simulink model "ALU_04_SS"  (R2022a)
settings: Solver=VariableStepAuto  StartTime=0.0  StopTime=10.0  RelTol=1e-3
undefined symbols (not defined in the file or in its folder): xc7z010iclg225
libraries: hdlBasic x1537, vmcUtilities x1
(part 3 of 8)

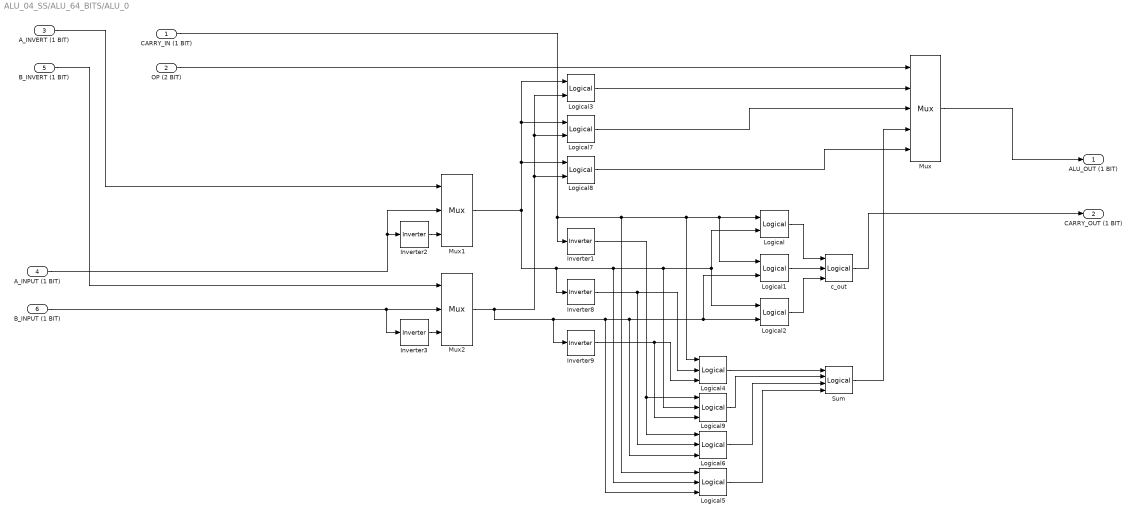
== system ALU_04_SS/ALU_64_BITS/ALU_0 ==
  CARRY_IN (1 BIT) : Inport
  OP (2 BIT) : Inport  Port=2
  A_INVERT (1 BIT) : Inport  Port=3
  A_INPUT (1 BIT) : Inport  Port=4
  B_INVERT (1 BIT) : Inport  Port=5
  B_INPUT (1 BIT) : Inport  Port=6
  Inverter{1..3,8..9} (5 alike) : hdlBasic/Inverter  en=off  latency=0  XmcBlockStatus=1  maskContainerNames=group2  block_type=inv  block_config=sysgen:Inverter_config
  Logical{,1..3} (4 alike) : hdlBasic/Logical  logical_function=AND  inputs=2  en=off  latency=0  precision=Full  arith_type=Unsigned  n_bits=16  bin_pt=0  align_bp=on  overflow=[]  quantization=[]  XmcBlockStatus=1  maskContainerNames=tabcontainer1  block_type=logical  block_config=sysgen:Logical_config
  Logical{4..6,9} (4 alike) : hdlBasic/Logical  logical_function=AND  inputs=3  en=off  latency=0  precision=Full  arith_type=Unsigned  n_bits=16  bin_pt=0  align_bp=on  overflow=[]  quantization=[]  XmcBlockStatus=1  maskContainerNames=tabcontainer1  block_type=logical  block_config=sysgen:Logical_config
  Logical7 : hdlBasic/Logical  logical_function=OR  inputs=2  en=off  latency=0  precision=Full  arith_type=Unsigned  n_bits=16  bin_pt=0  align_bp=on  overflow=[]  quantization=[]  XmcBlockStatus=1  maskContainerNames=tabcontainer1  block_type=logical  block_config=sysgen:Logical_config
  Logical8 : hdlBasic/Logical  logical_function=XOR  inputs=2  en=off  latency=0  precision=Full  arith_type=Unsigned  n_bits=16  bin_pt=0  align_bp=on  overflow=[]  quantization=[]  XmcBlockStatus=1  maskContainerNames=tabcontainer1  block_type=logical  block_config=sysgen:Logical_config
  Mux : hdlBasic/Mux  inputs=4  en=off  latency=0  precision=Full  arith_type=Unsigned  n_bits=16  bin_pt=14  quantization=Truncate  overflow=Wrap  XmcBlockStatus=1  maskContainerNames=tabcontainer1  block_type=mux  block_config=sysgen:Mux_config
  Mux1 : hdlBasic/Mux  inputs=2  en=off  latency=0  precision=Full  arith_type=Unsigned  n_bits=16  bin_pt=14  quantization=Truncate  overflow=Wrap  XmcBlockStatus=1  maskContainerNames=tabcontainer1  block_type=mux  block_config=sysgen:Mux_config
  Mux2 : hdlBasic/Mux  inputs=2  en=off  latency=0  precision=Full  arith_type=Unsigned  n_bits=16  bin_pt=14  quantization=Truncate  overflow=Wrap  XmcBlockStatus=1  maskContainerNames=tabcontainer1  block_type=mux  block_config=sysgen:Mux_config
  Sum : hdlBasic/Logical  logical_function=OR  inputs=4  en=off  latency=0  precision=Full  arith_type=Unsigned  n_bits=16  bin_pt=0  align_bp=on  overflow=[]  quantization=[]  XmcBlockStatus=1  maskContainerNames=tabcontainer1  block_type=logical  block_config=sysgen:Logical_config
  c_out : hdlBasic/Logical  logical_function=OR  inputs=3  en=off  latency=0  precision=Full  arith_type=Unsigned  n_bits=16  bin_pt=0  align_bp=on  overflow=[]  quantization=[]  XmcBlockStatus=1  maskContainerNames=tabcontainer1  block_type=logical  block_config=sysgen:Logical_config
  ALU_OUT (1 BIT) : Outport
  CARRY_OUT (1 BIT) : Outport  Port=2
  wires:
  Logical2/1 -> c_out/3
  A_INVERT (1 BIT)/1 -> Mux1/1
  c_out/1 -> CARRY_OUT (1 BIT)/1
  Sum/1 -> Mux/4
  CARRY_IN (1 BIT)/1 -> Inverter1/1, Logical5/1, Logical4/1, Logical1/1, Logical/1
  Mux2/1 -> Logical5/3, Logical6/3, Logical1/2, Logical2/2, Inverter9/1, Logical8/2, Logical3/2, Logical7/2
  B_INPUT (1 BIT)/1 -> Inverter3/1, Mux2/2
  Mux/1 -> ALU_OUT (1 BIT)/1
  Logical/1 -> c_out/1
  B_INVERT (1 BIT)/1 -> Mux2/1
  Logical6/1 -> Sum/3
  Mux1/1 -> Logical8/1, Logical7/1, Logical3/1, Inverter8/1, Logical5/2, Logical/2, Logical2/1, Logical9/2
  Logical5/1 -> Sum/4
  OP (2 BIT)/1 -> Mux/1
  Logical9/1 -> Sum/2
  Inverter1/1 -> Logical6/1, Logical9/1
  Inverter3/1 -> Mux2/3
  Inverter9/1 -> Logical9/3, Logical4/3
  A_INPUT (1 BIT)/1 -> Mux1/2, Inverter2/1
  Inverter2/1 -> Mux1/3
  Logical4/1 -> Sum/1
  Inverter8/1 -> Logical6/2, Logical4/2
  Logical3/1 -> Mux/2
  Logical7/1 -> Mux/3
  Logical1/1 -> c_out/2
  Logical8/1 -> Mux/5

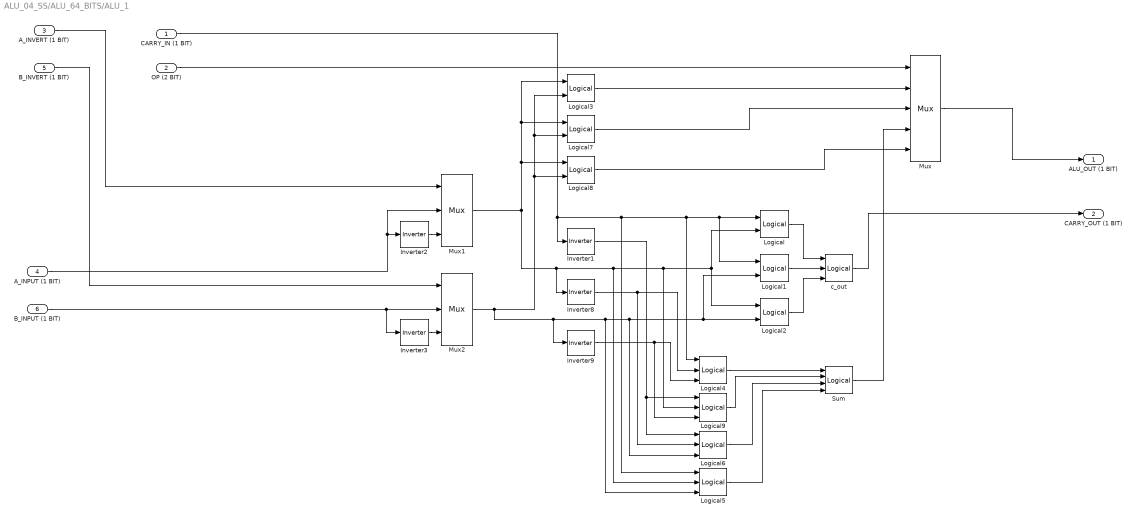
== system ALU_04_SS/ALU_64_BITS/ALU_1 ==
  CARRY_IN (1 BIT) : Inport
  OP (2 BIT) : Inport  Port=2
  A_INVERT (1 BIT) : Inport  Port=3
  A_INPUT (1 BIT) : Inport  Port=4
  B_INVERT (1 BIT) : Inport  Port=5
  B_INPUT (1 BIT) : Inport  Port=6
  Inverter{1..3,8..9} (5 alike) : hdlBasic/Inverter  en=off  latency=0  XmcBlockStatus=1  maskContainerNames=group2  block_type=inv  block_config=sysgen:Inverter_config
  Logical{,1..3} (4 alike) : hdlBasic/Logical  logical_function=AND  inputs=2  en=off  latency=0  precision=Full  arith_type=Unsigned  n_bits=16  bin_pt=0  align_bp=on  overflow=[]  quantization=[]  XmcBlockStatus=1  maskContainerNames=tabcontainer1  block_type=logical  block_config=sysgen:Logical_config
  Logical{4..6,9} (4 alike) : hdlBasic/Logical  logical_function=AND  inputs=3  en=off  latency=0  precision=Full  arith_type=Unsigned  n_bits=16  bin_pt=0  align_bp=on  overflow=[]  quantization=[]  XmcBlockStatus=1  maskContainerNames=tabcontainer1  block_type=logical  block_config=sysgen:Logical_config
  Logical7 : hdlBasic/Logical  logical_function=OR  inputs=2  en=off  latency=0  precision=Full  arith_type=Unsigned  n_bits=16  bin_pt=0  align_bp=on  overflow=[]  quantization=[]  XmcBlockStatus=1  maskContainerNames=tabcontainer1  block_type=logical  block_config=sysgen:Logical_config
  Logical8 : hdlBasic/Logical  logical_function=XOR  inputs=2  en=off  latency=0  precision=Full  arith_type=Unsigned  n_bits=16  bin_pt=0  align_bp=on  overflow=[]  quantization=[]  XmcBlockStatus=1  maskContainerNames=tabcontainer1  block_type=logical  block_config=sysgen:Logical_config
  Mux : hdlBasic/Mux  inputs=4  en=off  latency=0  precision=Full  arith_type=Unsigned  n_bits=16  bin_pt=14  quantization=Truncate  overflow=Wrap  XmcBlockStatus=1  maskContainerNames=tabcontainer1  block_type=mux  block_config=sysgen:Mux_config
  Mux1 : hdlBasic/Mux  inputs=2  en=off  latency=0  precision=Full  arith_type=Unsigned  n_bits=16  bin_pt=14  quantization=Truncate  overflow=Wrap  XmcBlockStatus=1  maskContainerNames=tabcontainer1  block_type=mux  block_config=sysgen:Mux_config
  Mux2 : hdlBasic/Mux  inputs=2  en=off  latency=0  precision=Full  arith_type=Unsigned  n_bits=16  bin_pt=14  quantization=Truncate  overflow=Wrap  XmcBlockStatus=1  maskContainerNames=tabcontainer1  block_type=mux  block_config=sysgen:Mux_config
  Sum : hdlBasic/Logical  logical_function=OR  inputs=4  en=off  latency=0  precision=Full  arith_type=Unsigned  n_bits=16  bin_pt=0  align_bp=on  overflow=[]  quantization=[]  XmcBlockStatus=1  maskContainerNames=tabcontainer1  block_type=logical  block_config=sysgen:Logical_config
  c_out : hdlBasic/Logical  logical_function=OR  inputs=3  en=off  latency=0  precision=Full  arith_type=Unsigned  n_bits=16  bin_pt=0  align_bp=on  overflow=[]  quantization=[]  XmcBlockStatus=1  maskContainerNames=tabcontainer1  block_type=logical  block_config=sysgen:Logical_config
  ALU_OUT (1 BIT) : Outport
  CARRY_OUT (1 BIT) : Outport  Port=2
  wires:
  Logical2/1 -> c_out/3
  A_INVERT (1 BIT)/1 -> Mux1/1
  c_out/1 -> CARRY_OUT (1 BIT)/1
  Sum/1 -> Mux/4
  CARRY_IN (1 BIT)/1 -> Inverter1/1, Logical5/1, Logical4/1, Logical1/1, Logical/1
  Mux2/1 -> Logical5/3, Logical6/3, Logical1/2, Logical2/2, Inverter9/1, Logical8/2, Logical3/2, Logical7/2
  B_INPUT (1 BIT)/1 -> Inverter3/1, Mux2/2
  Mux/1 -> ALU_OUT (1 BIT)/1
  Logical/1 -> c_out/1
  B_INVERT (1 BIT)/1 -> Mux2/1
  Logical6/1 -> Sum/3
  Mux1/1 -> Logical8/1, Logical7/1, Logical3/1, Inverter8/1, Logical5/2, Logical/2, Logical2/1, Logical9/2
  Logical5/1 -> Sum/4
  OP (2 BIT)/1 -> Mux/1
  Logical9/1 -> Sum/2
  Inverter1/1 -> Logical6/1, Logical9/1
  Inverter3/1 -> Mux2/3
  Inverter9/1 -> Logical9/3, Logical4/3
  A_INPUT (1 BIT)/1 -> Mux1/2, Inverter2/1
  Inverter2/1 -> Mux1/3
  Logical4/1 -> Sum/1
  Inverter8/1 -> Logical6/2, Logical4/2
  Logical3/1 -> Mux/2
  Logical7/1 -> Mux/3
  Logical1/1 -> c_out/2
  Logical8/1 -> Mux/5

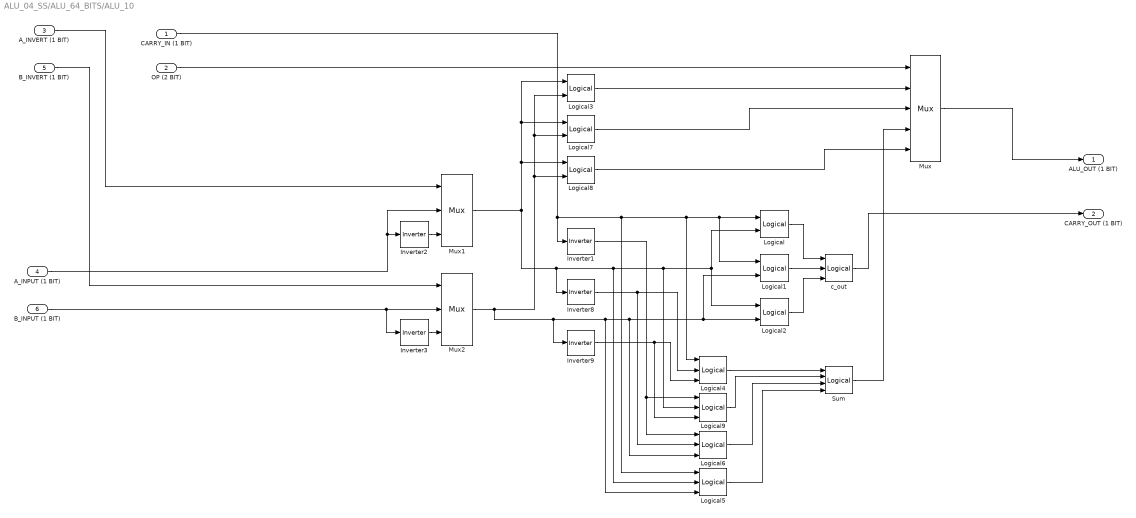
== system ALU_04_SS/ALU_64_BITS/ALU_10 ==
  CARRY_IN (1 BIT) : Inport
  OP (2 BIT) : Inport  Port=2
  A_INVERT (1 BIT) : Inport  Port=3
  A_INPUT (1 BIT) : Inport  Port=4
  B_INVERT (1 BIT) : Inport  Port=5
  B_INPUT (1 BIT) : Inport  Port=6
  Inverter{1..3,8..9} (5 alike) : hdlBasic/Inverter  en=off  latency=0  XmcBlockStatus=1  maskContainerNames=group2  block_type=inv  block_config=sysgen:Inverter_config
  Logical{,1..3} (4 alike) : hdlBasic/Logical  logical_function=AND  inputs=2  en=off  latency=0  precision=Full  arith_type=Unsigned  n_bits=16  bin_pt=0  align_bp=on  overflow=[]  quantization=[]  XmcBlockStatus=1  maskContainerNames=tabcontainer1  block_type=logical  block_config=sysgen:Logical_config
  Logical{4..6,9} (4 alike) : hdlBasic/Logical  logical_function=AND  inputs=3  en=off  latency=0  precision=Full  arith_type=Unsigned  n_bits=16  bin_pt=0  align_bp=on  overflow=[]  quantization=[]  XmcBlockStatus=1  maskContainerNames=tabcontainer1  block_type=logical  block_config=sysgen:Logical_config
  Logical7 : hdlBasic/Logical  logical_function=OR  inputs=2  en=off  latency=0  precision=Full  arith_type=Unsigned  n_bits=16  bin_pt=0  align_bp=on  overflow=[]  quantization=[]  XmcBlockStatus=1  maskContainerNames=tabcontainer1  block_type=logical  block_config=sysgen:Logical_config
  Logical8 : hdlBasic/Logical  logical_function=XOR  inputs=2  en=off  latency=0  precision=Full  arith_type=Unsigned  n_bits=16  bin_pt=0  align_bp=on  overflow=[]  quantization=[]  XmcBlockStatus=1  maskContainerNames=tabcontainer1  block_type=logical  block_config=sysgen:Logical_config
  Mux : hdlBasic/Mux  inputs=4  en=off  latency=0  precision=Full  arith_type=Unsigned  n_bits=16  bin_pt=14  quantization=Truncate  overflow=Wrap  XmcBlockStatus=1  maskContainerNames=tabcontainer1  block_type=mux  block_config=sysgen:Mux_config
  Mux1 : hdlBasic/Mux  inputs=2  en=off  latency=0  precision=Full  arith_type=Unsigned  n_bits=16  bin_pt=14  quantization=Truncate  overflow=Wrap  XmcBlockStatus=1  maskContainerNames=tabcontainer1  block_type=mux  block_config=sysgen:Mux_config
  Mux2 : hdlBasic/Mux  inputs=2  en=off  latency=0  precision=Full  arith_type=Unsigned  n_bits=16  bin_pt=14  quantization=Truncate  overflow=Wrap  XmcBlockStatus=1  maskContainerNames=tabcontainer1  block_type=mux  block_config=sysgen:Mux_config
  Sum : hdlBasic/Logical  logical_function=OR  inputs=4  en=off  latency=0  precision=Full  arith_type=Unsigned  n_bits=16  bin_pt=0  align_bp=on  overflow=[]  quantization=[]  XmcBlockStatus=1  maskContainerNames=tabcontainer1  block_type=logical  block_config=sysgen:Logical_config
  c_out : hdlBasic/Logical  logical_function=OR  inputs=3  en=off  latency=0  precision=Full  arith_type=Unsigned  n_bits=16  bin_pt=0  align_bp=on  overflow=[]  quantization=[]  XmcBlockStatus=1  maskContainerNames=tabcontainer1  block_type=logical  block_config=sysgen:Logical_config
  ALU_OUT (1 BIT) : Outport
  CARRY_OUT (1 BIT) : Outport  Port=2
  wires:
  Logical2/1 -> c_out/3
  A_INVERT (1 BIT)/1 -> Mux1/1
  c_out/1 -> CARRY_OUT (1 BIT)/1
  Sum/1 -> Mux/4
  CARRY_IN (1 BIT)/1 -> Inverter1/1, Logical5/1, Logical4/1, Logical1/1, Logical/1
  Mux2/1 -> Logical5/3, Logical6/3, Logical1/2, Logical2/2, Inverter9/1, Logical8/2, Logical3/2, Logical7/2
  B_INPUT (1 BIT)/1 -> Inverter3/1, Mux2/2
  Mux/1 -> ALU_OUT (1 BIT)/1
  Logical/1 -> c_out/1
  B_INVERT (1 BIT)/1 -> Mux2/1
  Logical6/1 -> Sum/3
  Mux1/1 -> Logical8/1, Logical7/1, Logical3/1, Inverter8/1, Logical5/2, Logical/2, Logical2/1, Logical9/2
  Logical5/1 -> Sum/4
  OP (2 BIT)/1 -> Mux/1
  Logical9/1 -> Sum/2
  Inverter1/1 -> Logical6/1, Logical9/1
  Inverter3/1 -> Mux2/3
  Inverter9/1 -> Logical9/3, Logical4/3
  A_INPUT (1 BIT)/1 -> Mux1/2, Inverter2/1
  Inverter2/1 -> Mux1/3
  Logical4/1 -> Sum/1
  Inverter8/1 -> Logical6/2, Logical4/2
  Logical3/1 -> Mux/2
  Logical7/1 -> Mux/3
  Logical1/1 -> c_out/2
  Logical8/1 -> Mux/5

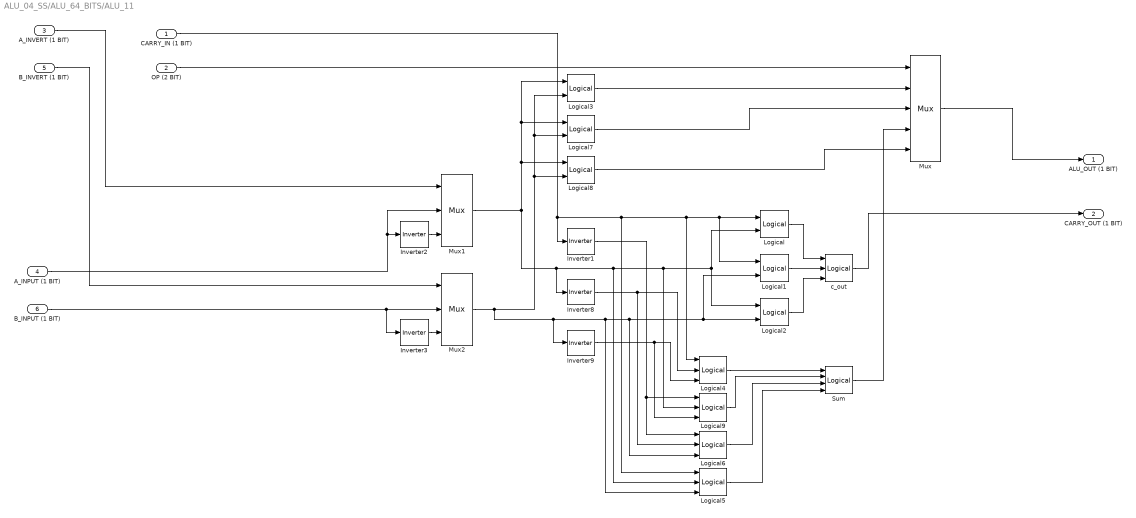
== system ALU_04_SS/ALU_64_BITS/ALU_11 ==
  CARRY_IN (1 BIT) : Inport
  OP (2 BIT) : Inport  Port=2
  A_INVERT (1 BIT) : Inport  Port=3
  A_INPUT (1 BIT) : Inport  Port=4
  B_INVERT (1 BIT) : Inport  Port=5
  B_INPUT (1 BIT) : Inport  Port=6
  Inverter{1..3,8..9} (5 alike) : hdlBasic/Inverter  en=off  latency=0  XmcBlockStatus=1  maskContainerNames=group2  block_type=inv  block_config=sysgen:Inverter_config
  Logical{,1..3} (4 alike) : hdlBasic/Logical  logical_function=AND  inputs=2  en=off  latency=0  precision=Full  arith_type=Unsigned  n_bits=16  bin_pt=0  align_bp=on  overflow=[]  quantization=[]  XmcBlockStatus=1  maskContainerNames=tabcontainer1  block_type=logical  block_config=sysgen:Logical_config
  Logical{4..6,9} (4 alike) : hdlBasic/Logical  logical_function=AND  inputs=3  en=off  latency=0  precision=Full  arith_type=Unsigned  n_bits=16  bin_pt=0  align_bp=on  overflow=[]  quantization=[]  XmcBlockStatus=1  maskContainerNames=tabcontainer1  block_type=logical  block_config=sysgen:Logical_config
  Logical7 : hdlBasic/Logical  logical_function=OR  inputs=2  en=off  latency=0  precision=Full  arith_type=Unsigned  n_bits=16  bin_pt=0  align_bp=on  overflow=[]  quantization=[]  XmcBlockStatus=1  maskContainerNames=tabcontainer1  block_type=logical  block_config=sysgen:Logical_config
  Logical8 : hdlBasic/Logical  logical_function=XOR  inputs=2  en=off  latency=0  precision=Full  arith_type=Unsigned  n_bits=16  bin_pt=0  align_bp=on  overflow=[]  quantization=[]  XmcBlockStatus=1  maskContainerNames=tabcontainer1  block_type=logical  block_config=sysgen:Logical_config
  Mux : hdlBasic/Mux  inputs=4  en=off  latency=0  precision=Full  arith_type=Unsigned  n_bits=16  bin_pt=14  quantization=Truncate  overflow=Wrap  XmcBlockStatus=1  maskContainerNames=tabcontainer1  block_type=mux  block_config=sysgen:Mux_config
  Mux1 : hdlBasic/Mux  inputs=2  en=off  latency=0  precision=Full  arith_type=Unsigned  n_bits=16  bin_pt=14  quantization=Truncate  overflow=Wrap  XmcBlockStatus=1  maskContainerNames=tabcontainer1  block_type=mux  block_config=sysgen:Mux_config
  Mux2 : hdlBasic/Mux  inputs=2  en=off  latency=0  precision=Full  arith_type=Unsigned  n_bits=16  bin_pt=14  quantization=Truncate  overflow=Wrap  XmcBlockStatus=1  maskContainerNames=tabcontainer1  block_type=mux  block_config=sysgen:Mux_config
  Sum : hdlBasic/Logical  logical_function=OR  inputs=4  en=off  latency=0  precision=Full  arith_type=Unsigned  n_bits=16  bin_pt=0  align_bp=on  overflow=[]  quantization=[]  XmcBlockStatus=1  maskContainerNames=tabcontainer1  block_type=logical  block_config=sysgen:Logical_config
  c_out : hdlBasic/Logical  logical_function=OR  inputs=3  en=off  latency=0  precision=Full  arith_type=Unsigned  n_bits=16  bin_pt=0  align_bp=on  overflow=[]  quantization=[]  XmcBlockStatus=1  maskContainerNames=tabcontainer1  block_type=logical  block_config=sysgen:Logical_config
  ALU_OUT (1 BIT) : Outport
  CARRY_OUT (1 BIT) : Outport  Port=2
  wires:
  Logical2/1 -> c_out/3
  A_INVERT (1 BIT)/1 -> Mux1/1
  c_out/1 -> CARRY_OUT (1 BIT)/1
  Sum/1 -> Mux/4
  CARRY_IN (1 BIT)/1 -> Inverter1/1, Logical5/1, Logical4/1, Logical1/1, Logical/1
  Mux2/1 -> Logical5/3, Logical6/3, Logical1/2, Logical2/2, Inverter9/1, Logical8/2, Logical3/2, Logical7/2
  B_INPUT (1 BIT)/1 -> Inverter3/1, Mux2/2
  Mux/1 -> ALU_OUT (1 BIT)/1
  Logical/1 -> c_out/1
  B_INVERT (1 BIT)/1 -> Mux2/1
  Logical6/1 -> Sum/3
  Mux1/1 -> Logical8/1, Logical7/1, Logical3/1, Inverter8/1, Logical5/2, Logical/2, Logical2/1, Logical9/2
  Logical5/1 -> Sum/4
  OP (2 BIT)/1 -> Mux/1
  Logical9/1 -> Sum/2
  Inverter1/1 -> Logical6/1, Logical9/1
  Inverter3/1 -> Mux2/3
  Inverter9/1 -> Logical9/3, Logical4/3
  A_INPUT (1 BIT)/1 -> Mux1/2, Inverter2/1
  Inverter2/1 -> Mux1/3
  Logical4/1 -> Sum/1
  Inverter8/1 -> Logical6/2, Logical4/2
  Logical3/1 -> Mux/2
  Logical7/1 -> Mux/3
  Logical1/1 -> c_out/2
  Logical8/1 -> Mux/5

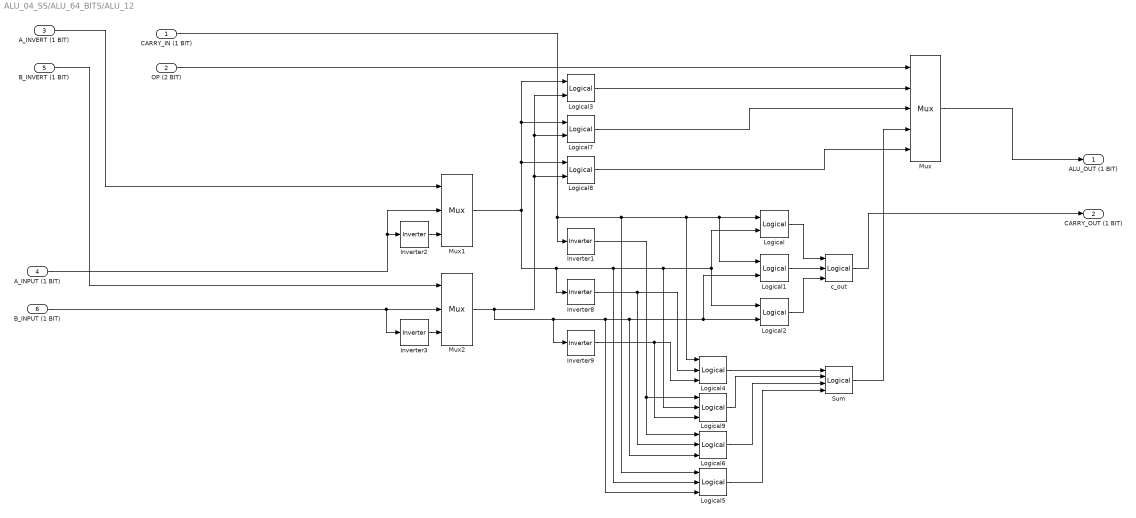
== system ALU_04_SS/ALU_64_BITS/ALU_12 ==
  CARRY_IN (1 BIT) : Inport
  OP (2 BIT) : Inport  Port=2
  A_INVERT (1 BIT) : Inport  Port=3
  A_INPUT (1 BIT) : Inport  Port=4
  B_INVERT (1 BIT) : Inport  Port=5
  B_INPUT (1 BIT) : Inport  Port=6
  Inverter{1..3,8..9} (5 alike) : hdlBasic/Inverter  en=off  latency=0  XmcBlockStatus=1  maskContainerNames=group2  block_type=inv  block_config=sysgen:Inverter_config
  Logical{,1..3} (4 alike) : hdlBasic/Logical  logical_function=AND  inputs=2  en=off  latency=0  precision=Full  arith_type=Unsigned  n_bits=16  bin_pt=0  align_bp=on  overflow=[]  quantization=[]  XmcBlockStatus=1  maskContainerNames=tabcontainer1  block_type=logical  block_config=sysgen:Logical_config
  Logical{4..6,9} (4 alike) : hdlBasic/Logical  logical_function=AND  inputs=3  en=off  latency=0  precision=Full  arith_type=Unsigned  n_bits=16  bin_pt=0  align_bp=on  overflow=[]  quantization=[]  XmcBlockStatus=1  maskContainerNames=tabcontainer1  block_type=logical  block_config=sysgen:Logical_config
  Logical7 : hdlBasic/Logical  logical_function=OR  inputs=2  en=off  latency=0  precision=Full  arith_type=Unsigned  n_bits=16  bin_pt=0  align_bp=on  overflow=[]  quantization=[]  XmcBlockStatus=1  maskContainerNames=tabcontainer1  block_type=logical  block_config=sysgen:Logical_config
  Logical8 : hdlBasic/Logical  logical_function=XOR  inputs=2  en=off  latency=0  precision=Full  arith_type=Unsigned  n_bits=16  bin_pt=0  align_bp=on  overflow=[]  quantization=[]  XmcBlockStatus=1  maskContainerNames=tabcontainer1  block_type=logical  block_config=sysgen:Logical_config
  Mux : hdlBasic/Mux  inputs=4  en=off  latency=0  precision=Full  arith_type=Unsigned  n_bits=16  bin_pt=14  quantization=Truncate  overflow=Wrap  XmcBlockStatus=1  maskContainerNames=tabcontainer1  block_type=mux  block_config=sysgen:Mux_config
  Mux1 : hdlBasic/Mux  inputs=2  en=off  latency=0  precision=Full  arith_type=Unsigned  n_bits=16  bin_pt=14  quantization=Truncate  overflow=Wrap  XmcBlockStatus=1  maskContainerNames=tabcontainer1  block_type=mux  block_config=sysgen:Mux_config
  Mux2 : hdlBasic/Mux  inputs=2  en=off  latency=0  precision=Full  arith_type=Unsigned  n_bits=16  bin_pt=14  quantization=Truncate  overflow=Wrap  XmcBlockStatus=1  maskContainerNames=tabcontainer1  block_type=mux  block_config=sysgen:Mux_config
  Sum : hdlBasic/Logical  logical_function=OR  inputs=4  en=off  latency=0  precision=Full  arith_type=Unsigned  n_bits=16  bin_pt=0  align_bp=on  overflow=[]  quantization=[]  XmcBlockStatus=1  maskContainerNames=tabcontainer1  block_type=logical  block_config=sysgen:Logical_config
  c_out : hdlBasic/Logical  logical_function=OR  inputs=3  en=off  latency=0  precision=Full  arith_type=Unsigned  n_bits=16  bin_pt=0  align_bp=on  overflow=[]  quantization=[]  XmcBlockStatus=1  maskContainerNames=tabcontainer1  block_type=logical  block_config=sysgen:Logical_config
  ALU_OUT (1 BIT) : Outport
  CARRY_OUT (1 BIT) : Outport  Port=2
  wires:
  Logical2/1 -> c_out/3
  A_INVERT (1 BIT)/1 -> Mux1/1
  c_out/1 -> CARRY_OUT (1 BIT)/1
  Sum/1 -> Mux/4
  CARRY_IN (1 BIT)/1 -> Inverter1/1, Logical5/1, Logical4/1, Logical1/1, Logical/1
  Mux2/1 -> Logical5/3, Logical6/3, Logical1/2, Logical2/2, Inverter9/1, Logical8/2, Logical3/2, Logical7/2
  B_INPUT (1 BIT)/1 -> Inverter3/1, Mux2/2
  Mux/1 -> ALU_OUT (1 BIT)/1
  Logical/1 -> c_out/1
  B_INVERT (1 BIT)/1 -> Mux2/1
  Logical6/1 -> Sum/3
  Mux1/1 -> Logical8/1, Logical7/1, Logical3/1, Inverter8/1, Logical5/2, Logical/2, Logical2/1, Logical9/2
  Logical5/1 -> Sum/4
  OP (2 BIT)/1 -> Mux/1
  Logical9/1 -> Sum/2
  Inverter1/1 -> Logical6/1, Logical9/1
  Inverter3/1 -> Mux2/3
  Inverter9/1 -> Logical9/3, Logical4/3
  A_INPUT (1 BIT)/1 -> Mux1/2, Inverter2/1
  Inverter2/1 -> Mux1/3
  Logical4/1 -> Sum/1
  Inverter8/1 -> Logical6/2, Logical4/2
  Logical3/1 -> Mux/2
  Logical7/1 -> Mux/3
  Logical1/1 -> c_out/2
  Logical8/1 -> Mux/5

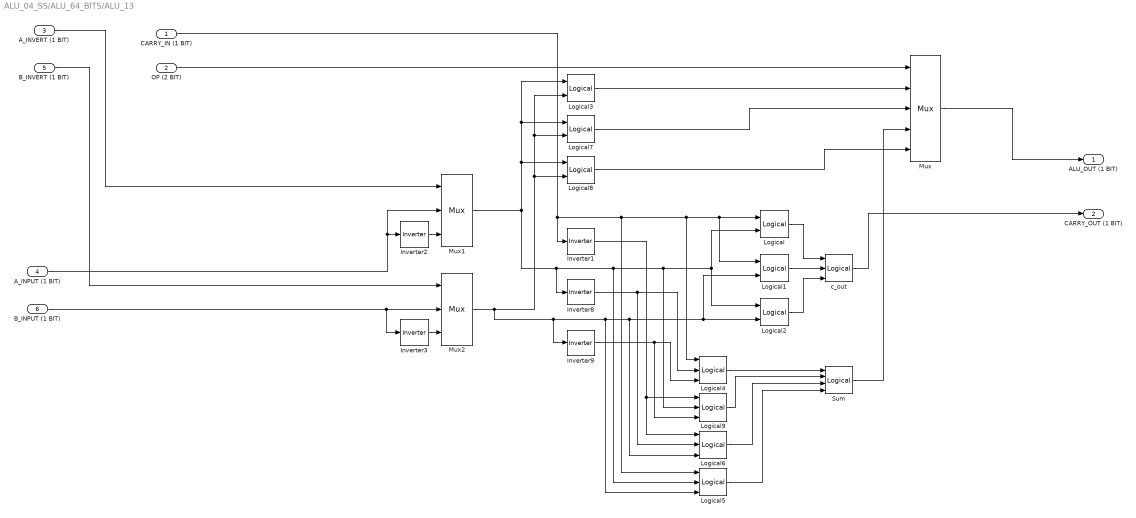
== system ALU_04_SS/ALU_64_BITS/ALU_13 ==
  CARRY_IN (1 BIT) : Inport
  OP (2 BIT) : Inport  Port=2
  A_INVERT (1 BIT) : Inport  Port=3
  A_INPUT (1 BIT) : Inport  Port=4
  B_INVERT (1 BIT) : Inport  Port=5
  B_INPUT (1 BIT) : Inport  Port=6
  Inverter{1..3,8..9} (5 alike) : hdlBasic/Inverter  en=off  latency=0  XmcBlockStatus=1  maskContainerNames=group2  block_type=inv  block_config=sysgen:Inverter_config
  Logical{,1..3} (4 alike) : hdlBasic/Logical  logical_function=AND  inputs=2  en=off  latency=0  precision=Full  arith_type=Unsigned  n_bits=16  bin_pt=0  align_bp=on  overflow=[]  quantization=[]  XmcBlockStatus=1  maskContainerNames=tabcontainer1  block_type=logical  block_config=sysgen:Logical_config
  Logical{4..6,9} (4 alike) : hdlBasic/Logical  logical_function=AND  inputs=3  en=off  latency=0  precision=Full  arith_type=Unsigned  n_bits=16  bin_pt=0  align_bp=on  overflow=[]  quantization=[]  XmcBlockStatus=1  maskContainerNames=tabcontainer1  block_type=logical  block_config=sysgen:Logical_config
  Logical7 : hdlBasic/Logical  logical_function=OR  inputs=2  en=off  latency=0  precision=Full  arith_type=Unsigned  n_bits=16  bin_pt=0  align_bp=on  overflow=[]  quantization=[]  XmcBlockStatus=1  maskContainerNames=tabcontainer1  block_type=logical  block_config=sysgen:Logical_config
  Logical8 : hdlBasic/Logical  logical_function=XOR  inputs=2  en=off  latency=0  precision=Full  arith_type=Unsigned  n_bits=16  bin_pt=0  align_bp=on  overflow=[]  quantization=[]  XmcBlockStatus=1  maskContainerNames=tabcontainer1  block_type=logical  block_config=sysgen:Logical_config
  Mux : hdlBasic/Mux  inputs=4  en=off  latency=0  precision=Full  arith_type=Unsigned  n_bits=16  bin_pt=14  quantization=Truncate  overflow=Wrap  XmcBlockStatus=1  maskContainerNames=tabcontainer1  block_type=mux  block_config=sysgen:Mux_config
  Mux1 : hdlBasic/Mux  inputs=2  en=off  latency=0  precision=Full  arith_type=Unsigned  n_bits=16  bin_pt=14  quantization=Truncate  overflow=Wrap  XmcBlockStatus=1  maskContainerNames=tabcontainer1  block_type=mux  block_config=sysgen:Mux_config
  Mux2 : hdlBasic/Mux  inputs=2  en=off  latency=0  precision=Full  arith_type=Unsigned  n_bits=16  bin_pt=14  quantization=Truncate  overflow=Wrap  XmcBlockStatus=1  maskContainerNames=tabcontainer1  block_type=mux  block_config=sysgen:Mux_config
  Sum : hdlBasic/Logical  logical_function=OR  inputs=4  en=off  latency=0  precision=Full  arith_type=Unsigned  n_bits=16  bin_pt=0  align_bp=on  overflow=[]  quantization=[]  XmcBlockStatus=1  maskContainerNames=tabcontainer1  block_type=logical  block_config=sysgen:Logical_config
  c_out : hdlBasic/Logical  logical_function=OR  inputs=3  en=off  latency=0  precision=Full  arith_type=Unsigned  n_bits=16  bin_pt=0  align_bp=on  overflow=[]  quantization=[]  XmcBlockStatus=1  maskContainerNames=tabcontainer1  block_type=logical  block_config=sysgen:Logical_config
  ALU_OUT (1 BIT) : Outport
  CARRY_OUT (1 BIT) : Outport  Port=2
  wires:
  Logical2/1 -> c_out/3
  A_INVERT (1 BIT)/1 -> Mux1/1
  c_out/1 -> CARRY_OUT (1 BIT)/1
  Sum/1 -> Mux/4
  CARRY_IN (1 BIT)/1 -> Inverter1/1, Logical5/1, Logical4/1, Logical1/1, Logical/1
  Mux2/1 -> Logical5/3, Logical6/3, Logical1/2, Logical2/2, Inverter9/1, Logical8/2, Logical3/2, Logical7/2
  B_INPUT (1 BIT)/1 -> Inverter3/1, Mux2/2
  Mux/1 -> ALU_OUT (1 BIT)/1
  Logical/1 -> c_out/1
  B_INVERT (1 BIT)/1 -> Mux2/1
  Logical6/1 -> Sum/3
  Mux1/1 -> Logical8/1, Logical7/1, Logical3/1, Inverter8/1, Logical5/2, Logical/2, Logical2/1, Logical9/2
  Logical5/1 -> Sum/4
  OP (2 BIT)/1 -> Mux/1
  Logical9/1 -> Sum/2
  Inverter1/1 -> Logical6/1, Logical9/1
  Inverter3/1 -> Mux2/3
  Inverter9/1 -> Logical9/3, Logical4/3
  A_INPUT (1 BIT)/1 -> Mux1/2, Inverter2/1
  Inverter2/1 -> Mux1/3
  Logical4/1 -> Sum/1
  Inverter8/1 -> Logical6/2, Logical4/2
  Logical3/1 -> Mux/2
  Logical7/1 -> Mux/3
  Logical1/1 -> c_out/2
  Logical8/1 -> Mux/5

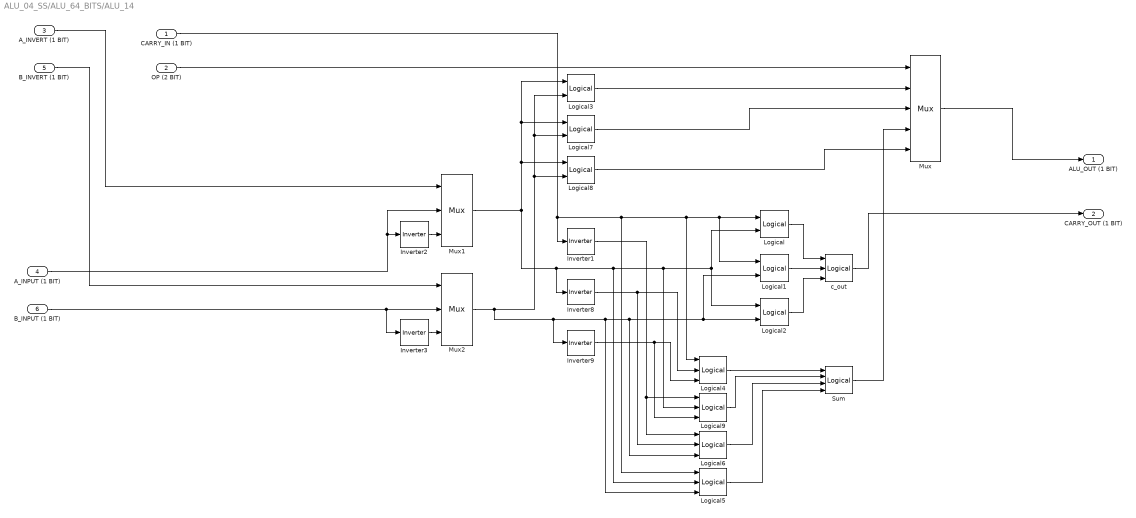
== system ALU_04_SS/ALU_64_BITS/ALU_14 ==
  CARRY_IN (1 BIT) : Inport
  OP (2 BIT) : Inport  Port=2
  A_INVERT (1 BIT) : Inport  Port=3
  A_INPUT (1 BIT) : Inport  Port=4
  B_INVERT (1 BIT) : Inport  Port=5
  B_INPUT (1 BIT) : Inport  Port=6
  Inverter{1..3,8..9} (5 alike) : hdlBasic/Inverter  en=off  latency=0  XmcBlockStatus=1  maskContainerNames=group2  block_type=inv  block_config=sysgen:Inverter_config
  Logical{,1..3} (4 alike) : hdlBasic/Logical  logical_function=AND  inputs=2  en=off  latency=0  precision=Full  arith_type=Unsigned  n_bits=16  bin_pt=0  align_bp=on  overflow=[]  quantization=[]  XmcBlockStatus=1  maskContainerNames=tabcontainer1  block_type=logical  block_config=sysgen:Logical_config
  Logical{4..6,9} (4 alike) : hdlBasic/Logical  logical_function=AND  inputs=3  en=off  latency=0  precision=Full  arith_type=Unsigned  n_bits=16  bin_pt=0  align_bp=on  overflow=[]  quantization=[]  XmcBlockStatus=1  maskContainerNames=tabcontainer1  block_type=logical  block_config=sysgen:Logical_config
  Logical7 : hdlBasic/Logical  logical_function=OR  inputs=2  en=off  latency=0  precision=Full  arith_type=Unsigned  n_bits=16  bin_pt=0  align_bp=on  overflow=[]  quantization=[]  XmcBlockStatus=1  maskContainerNames=tabcontainer1  block_type=logical  block_config=sysgen:Logical_config
  Logical8 : hdlBasic/Logical  logical_function=XOR  inputs=2  en=off  latency=0  precision=Full  arith_type=Unsigned  n_bits=16  bin_pt=0  align_bp=on  overflow=[]  quantization=[]  XmcBlockStatus=1  maskContainerNames=tabcontainer1  block_type=logical  block_config=sysgen:Logical_config
  Mux : hdlBasic/Mux  inputs=4  en=off  latency=0  precision=Full  arith_type=Unsigned  n_bits=16  bin_pt=14  quantization=Truncate  overflow=Wrap  XmcBlockStatus=1  maskContainerNames=tabcontainer1  block_type=mux  block_config=sysgen:Mux_config
  Mux1 : hdlBasic/Mux  inputs=2  en=off  latency=0  precision=Full  arith_type=Unsigned  n_bits=16  bin_pt=14  quantization=Truncate  overflow=Wrap  XmcBlockStatus=1  maskContainerNames=tabcontainer1  block_type=mux  block_config=sysgen:Mux_config
  Mux2 : hdlBasic/Mux  inputs=2  en=off  latency=0  precision=Full  arith_type=Unsigned  n_bits=16  bin_pt=14  quantization=Truncate  overflow=Wrap  XmcBlockStatus=1  maskContainerNames=tabcontainer1  block_type=mux  block_config=sysgen:Mux_config
  Sum : hdlBasic/Logical  logical_function=OR  inputs=4  en=off  latency=0  precision=Full  arith_type=Unsigned  n_bits=16  bin_pt=0  align_bp=on  overflow=[]  quantization=[]  XmcBlockStatus=1  maskContainerNames=tabcontainer1  block_type=logical  block_config=sysgen:Logical_config
  c_out : hdlBasic/Logical  logical_function=OR  inputs=3  en=off  latency=0  precision=Full  arith_type=Unsigned  n_bits=16  bin_pt=0  align_bp=on  overflow=[]  quantization=[]  XmcBlockStatus=1  maskContainerNames=tabcontainer1  block_type=logical  block_config=sysgen:Logical_config
  ALU_OUT (1 BIT) : Outport
  CARRY_OUT (1 BIT) : Outport  Port=2
  wires:
  Logical2/1 -> c_out/3
  A_INVERT (1 BIT)/1 -> Mux1/1
  c_out/1 -> CARRY_OUT (1 BIT)/1
  Sum/1 -> Mux/4
  CARRY_IN (1 BIT)/1 -> Inverter1/1, Logical5/1, Logical4/1, Logical1/1, Logical/1
  Mux2/1 -> Logical5/3, Logical6/3, Logical1/2, Logical2/2, Inverter9/1, Logical8/2, Logical3/2, Logical7/2
  B_INPUT (1 BIT)/1 -> Inverter3/1, Mux2/2
  Mux/1 -> ALU_OUT (1 BIT)/1
  Logical/1 -> c_out/1
  B_INVERT (1 BIT)/1 -> Mux2/1
  Logical6/1 -> Sum/3
  Mux1/1 -> Logical8/1, Logical7/1, Logical3/1, Inverter8/1, Logical5/2, Logical/2, Logical2/1, Logical9/2
  Logical5/1 -> Sum/4
  OP (2 BIT)/1 -> Mux/1
  Logical9/1 -> Sum/2
  Inverter1/1 -> Logical6/1, Logical9/1
  Inverter3/1 -> Mux2/3
  Inverter9/1 -> Logical9/3, Logical4/3
  A_INPUT (1 BIT)/1 -> Mux1/2, Inverter2/1
  Inverter2/1 -> Mux1/3
  Logical4/1 -> Sum/1
  Inverter8/1 -> Logical6/2, Logical4/2
  Logical3/1 -> Mux/2
  Logical7/1 -> Mux/3
  Logical1/1 -> c_out/2
  Logical8/1 -> Mux/5

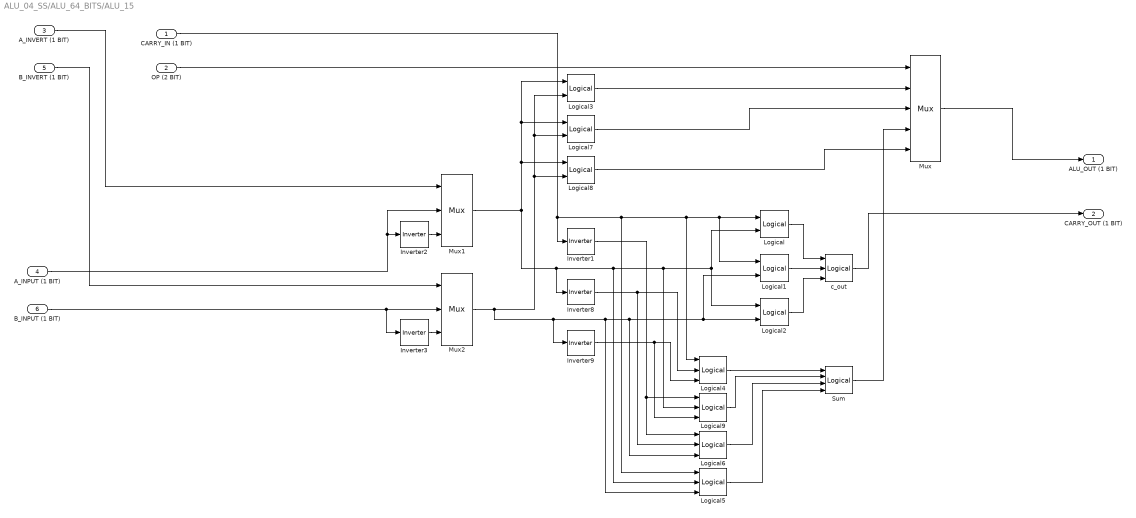
== system ALU_04_SS/ALU_64_BITS/ALU_15 ==
  CARRY_IN (1 BIT) : Inport
  OP (2 BIT) : Inport  Port=2
  A_INVERT (1 BIT) : Inport  Port=3
  A_INPUT (1 BIT) : Inport  Port=4
  B_INVERT (1 BIT) : Inport  Port=5
  B_INPUT (1 BIT) : Inport  Port=6
  Inverter{1..3,8..9} (5 alike) : hdlBasic/Inverter  en=off  latency=0  XmcBlockStatus=1  maskContainerNames=group2  block_type=inv  block_config=sysgen:Inverter_config
  Logical{,1..3} (4 alike) : hdlBasic/Logical  logical_function=AND  inputs=2  en=off  latency=0  precision=Full  arith_type=Unsigned  n_bits=16  bin_pt=0  align_bp=on  overflow=[]  quantization=[]  XmcBlockStatus=1  maskContainerNames=tabcontainer1  block_type=logical  block_config=sysgen:Logical_config
  Logical{4..6,9} (4 alike) : hdlBasic/Logical  logical_function=AND  inputs=3  en=off  latency=0  precision=Full  arith_type=Unsigned  n_bits=16  bin_pt=0  align_bp=on  overflow=[]  quantization=[]  XmcBlockStatus=1  maskContainerNames=tabcontainer1  block_type=logical  block_config=sysgen:Logical_config
  Logical7 : hdlBasic/Logical  logical_function=OR  inputs=2  en=off  latency=0  precision=Full  arith_type=Unsigned  n_bits=16  bin_pt=0  align_bp=on  overflow=[]  quantization=[]  XmcBlockStatus=1  maskContainerNames=tabcontainer1  block_type=logical  block_config=sysgen:Logical_config
  Logical8 : hdlBasic/Logical  logical_function=XOR  inputs=2  en=off  latency=0  precision=Full  arith_type=Unsigned  n_bits=16  bin_pt=0  align_bp=on  overflow=[]  quantization=[]  XmcBlockStatus=1  maskContainerNames=tabcontainer1  block_type=logical  block_config=sysgen:Logical_config
  Mux : hdlBasic/Mux  inputs=4  en=off  latency=0  precision=Full  arith_type=Unsigned  n_bits=16  bin_pt=14  quantization=Truncate  overflow=Wrap  XmcBlockStatus=1  maskContainerNames=tabcontainer1  block_type=mux  block_config=sysgen:Mux_config
  Mux1 : hdlBasic/Mux  inputs=2  en=off  latency=0  precision=Full  arith_type=Unsigned  n_bits=16  bin_pt=14  quantization=Truncate  overflow=Wrap  XmcBlockStatus=1  maskContainerNames=tabcontainer1  block_type=mux  block_config=sysgen:Mux_config
  Mux2 : hdlBasic/Mux  inputs=2  en=off  latency=0  precision=Full  arith_type=Unsigned  n_bits=16  bin_pt=14  quantization=Truncate  overflow=Wrap  XmcBlockStatus=1  maskContainerNames=tabcontainer1  block_type=mux  block_config=sysgen:Mux_config
  Sum : hdlBasic/Logical  logical_function=OR  inputs=4  en=off  latency=0  precision=Full  arith_type=Unsigned  n_bits=16  bin_pt=0  align_bp=on  overflow=[]  quantization=[]  XmcBlockStatus=1  maskContainerNames=tabcontainer1  block_type=logical  block_config=sysgen:Logical_config
  c_out : hdlBasic/Logical  logical_function=OR  inputs=3  en=off  latency=0  precision=Full  arith_type=Unsigned  n_bits=16  bin_pt=0  align_bp=on  overflow=[]  quantization=[]  XmcBlockStatus=1  maskContainerNames=tabcontainer1  block_type=logical  block_config=sysgen:Logical_config
  ALU_OUT (1 BIT) : Outport
  CARRY_OUT (1 BIT) : Outport  Port=2
  wires:
  Logical2/1 -> c_out/3
  A_INVERT (1 BIT)/1 -> Mux1/1
  c_out/1 -> CARRY_OUT (1 BIT)/1
  Sum/1 -> Mux/4
  CARRY_IN (1 BIT)/1 -> Inverter1/1, Logical5/1, Logical4/1, Logical1/1, Logical/1
  Mux2/1 -> Logical5/3, Logical6/3, Logical1/2, Logical2/2, Inverter9/1, Logical8/2, Logical3/2, Logical7/2
  B_INPUT (1 BIT)/1 -> Inverter3/1, Mux2/2
  Mux/1 -> ALU_OUT (1 BIT)/1
  Logical/1 -> c_out/1
  B_INVERT (1 BIT)/1 -> Mux2/1
  Logical6/1 -> Sum/3
  Mux1/1 -> Logical8/1, Logical7/1, Logical3/1, Inverter8/1, Logical5/2, Logical/2, Logical2/1, Logical9/2
  Logical5/1 -> Sum/4
  OP (2 BIT)/1 -> Mux/1
  Logical9/1 -> Sum/2
  Inverter1/1 -> Logical6/1, Logical9/1
  Inverter3/1 -> Mux2/3
  Inverter9/1 -> Logical9/3, Logical4/3
  A_INPUT (1 BIT)/1 -> Mux1/2, Inverter2/1
  Inverter2/1 -> Mux1/3
  Logical4/1 -> Sum/1
  Inverter8/1 -> Logical6/2, Logical4/2
  Logical3/1 -> Mux/2
  Logical7/1 -> Mux/3
  Logical1/1 -> c_out/2
  Logical8/1 -> Mux/5

== system ALU_04_SS/ALU_64_BITS/ALU_16 ==
  CARRY_IN (1 BIT) : Inport
  OP (2 BIT) : Inport  Port=2
  A_INVERT (1 BIT) : Inport  Port=3
  A_INPUT (1 BIT) : Inport  Port=4
  B_INVERT (1 BIT) : Inport  Port=5
  B_INPUT (1 BIT) : Inport  Port=6
  Inverter{1..3,8..9} (5 alike) : hdlBasic/Inverter  en=off  latency=0  XmcBlockStatus=1  maskContainerNames=group2  block_type=inv  block_config=sysgen:Inverter_config
  Logical{,1..3} (4 alike) : hdlBasic/Logical  logical_function=AND  inputs=2  en=off  latency=0  precision=Full  arith_type=Unsigned  n_bits=16  bin_pt=0  align_bp=on  overflow=[]  quantization=[]  XmcBlockStatus=1  maskContainerNames=tabcontainer1  block_type=logical  block_config=sysgen:Logical_config
  Logical{4..6,9} (4 alike) : hdlBasic/Logical  logical_function=AND  inputs=3  en=off  latency=0  precision=Full  arith_type=Unsigned  n_bits=16  bin_pt=0  align_bp=on  overflow=[]  quantization=[]  XmcBlockStatus=1  maskContainerNames=tabcontainer1  block_type=logical  block_config=sysgen:Logical_config
  Logical7 : hdlBasic/Logical  logical_function=OR  inputs=2  en=off  latency=0  precision=Full  arith_type=Unsigned  n_bits=16  bin_pt=0  align_bp=on  overflow=[]  quantization=[]  XmcBlockStatus=1  maskContainerNames=tabcontainer1  block_type=logical  block_config=sysgen:Logical_config
  Logical8 : hdlBasic/Logical  logical_function=XOR  inputs=2  en=off  latency=0  precision=Full  arith_type=Unsigned  n_bits=16  bin_pt=0  align_bp=on  overflow=[]  quantization=[]  XmcBlockStatus=1  maskContainerNames=tabcontainer1  block_type=logical  block_config=sysgen:Logical_config
  Mux : hdlBasic/Mux  inputs=4  en=off  latency=0  precision=Full  arith_type=Unsigned  n_bits=16  bin_pt=14  quantization=Truncate  overflow=Wrap  XmcBlockStatus=1  maskContainerNames=tabcontainer1  block_type=mux  block_config=sysgen:Mux_config
  Mux1 : hdlBasic/Mux  inputs=2  en=off  latency=0  precision=Full  arith_type=Unsigned  n_bits=16  bin_pt=14  quantization=Truncate  overflow=Wrap  XmcBlockStatus=1  maskContainerNames=tabcontainer1  block_type=mux  block_config=sysgen:Mux_config
  Mux2 : hdlBasic/Mux  inputs=2  en=off  latency=0  precision=Full  arith_type=Unsigned  n_bits=16  bin_pt=14  quantization=Truncate  overflow=Wrap  XmcBlockStatus=1  maskContainerNames=tabcontainer1  block_type=mux  block_config=sysgen:Mux_config
  Sum : hdlBasic/Logical  logical_function=OR  inputs=4  en=off  latency=0  precision=Full  arith_type=Unsigned  n_bits=16  bin_pt=0  align_bp=on  overflow=[]  quantization=[]  XmcBlockStatus=1  maskContainerNames=tabcontainer1  block_type=logical  block_config=sysgen:Logical_config
  c_out : hdlBasic/Logical  logical_function=OR  inputs=3  en=off  latency=0  precision=Full  arith_type=Unsigned  n_bits=16  bin_pt=0  align_bp=on  overflow=[]  quantization=[]  XmcBlockStatus=1  maskContainerNames=tabcontainer1  block_type=logical  block_config=sysgen:Logical_config
  ALU_OUT (1 BIT) : Outport
  CARRY_OUT (1 BIT) : Outport  Port=2
  wires:
  Logical2/1 -> c_out/3
  A_INVERT (1 BIT)/1 -> Mux1/1
  c_out/1 -> CARRY_OUT (1 BIT)/1
  Sum/1 -> Mux/4
  CARRY_IN (1 BIT)/1 -> Inverter1/1, Logical5/1, Logical4/1, Logical1/1, Logical/1
  Mux2/1 -> Logical5/3, Logical6/3, Logical1/2, Logical2/2, Inverter9/1, Logical8/2, Logical3/2, Logical7/2
  B_INPUT (1 BIT)/1 -> Inverter3/1, Mux2/2
  Mux/1 -> ALU_OUT (1 BIT)/1
  Logical/1 -> c_out/1
  B_INVERT (1 BIT)/1 -> Mux2/1
  Logical6/1 -> Sum/3
  Mux1/1 -> Logical8/1, Logical7/1, Logical3/1, Inverter8/1, Logical5/2, Logical/2, Logical2/1, Logical9/2
  Logical5/1 -> Sum/4
  OP (2 BIT)/1 -> Mux/1
  Logical9/1 -> Sum/2
  Inverter1/1 -> Logical6/1, Logical9/1
  Inverter3/1 -> Mux2/3
  Inverter9/1 -> Logical9/3, Logical4/3
  A_INPUT (1 BIT)/1 -> Mux1/2, Inverter2/1
  Inverter2/1 -> Mux1/3
  Logical4/1 -> Sum/1
  Inverter8/1 -> Logical6/2, Logical4/2
  Logical3/1 -> Mux/2
  Logical7/1 -> Mux/3
  Logical1/1 -> c_out/2
  Logical8/1 -> Mux/5

== system ALU_04_SS/ALU_64_BITS/ALU_17 ==
  CARRY_IN (1 BIT) : Inport
  OP (2 BIT) : Inport  Port=2
  A_INVERT (1 BIT) : Inport  Port=3
  A_INPUT (1 BIT) : Inport  Port=4
  B_INVERT (1 BIT) : Inport  Port=5
  B_INPUT (1 BIT) : Inport  Port=6
  Inverter{1..3,8..9} (5 alike) : hdlBasic/Inverter  en=off  latency=0  XmcBlockStatus=1  maskContainerNames=group2  block_type=inv  block_config=sysgen:Inverter_config
  Logical{,1..3} (4 alike) : hdlBasic/Logical  logical_function=AND  inputs=2  en=off  latency=0  precision=Full  arith_type=Unsigned  n_bits=16  bin_pt=0  align_bp=on  overflow=[]  quantization=[]  XmcBlockStatus=1  maskContainerNames=tabcontainer1  block_type=logical  block_config=sysgen:Logical_config
  Logical{4..6,9} (4 alike) : hdlBasic/Logical  logical_function=AND  inputs=3  en=off  latency=0  precision=Full  arith_type=Unsigned  n_bits=16  bin_pt=0  align_bp=on  overflow=[]  quantization=[]  XmcBlockStatus=1  maskContainerNames=tabcontainer1  block_type=logical  block_config=sysgen:Logical_config
  Logical7 : hdlBasic/Logical  logical_function=OR  inputs=2  en=off  latency=0  precision=Full  arith_type=Unsigned  n_bits=16  bin_pt=0  align_bp=on  overflow=[]  quantization=[]  XmcBlockStatus=1  maskContainerNames=tabcontainer1  block_type=logical  block_config=sysgen:Logical_config
  Logical8 : hdlBasic/Logical  logical_function=XOR  inputs=2  en=off  latency=0  precision=Full  arith_type=Unsigned  n_bits=16  bin_pt=0  align_bp=on  overflow=[]  quantization=[]  XmcBlockStatus=1  maskContainerNames=tabcontainer1  block_type=logical  block_config=sysgen:Logical_config
  Mux : hdlBasic/Mux  inputs=4  en=off  latency=0  precision=Full  arith_type=Unsigned  n_bits=16  bin_pt=14  quantization=Truncate  overflow=Wrap  XmcBlockStatus=1  maskContainerNames=tabcontainer1  block_type=mux  block_config=sysgen:Mux_config
  Mux1 : hdlBasic/Mux  inputs=2  en=off  latency=0  precision=Full  arith_type=Unsigned  n_bits=16  bin_pt=14  quantization=Truncate  overflow=Wrap  XmcBlockStatus=1  maskContainerNames=tabcontainer1  block_type=mux  block_config=sysgen:Mux_config
  Mux2 : hdlBasic/Mux  inputs=2  en=off  latency=0  precision=Full  arith_type=Unsigned  n_bits=16  bin_pt=14  quantization=Truncate  overflow=Wrap  XmcBlockStatus=1  maskContainerNames=tabcontainer1  block_type=mux  block_config=sysgen:Mux_config
  Sum : hdlBasic/Logical  logical_function=OR  inputs=4  en=off  latency=0  precision=Full  arith_type=Unsigned  n_bits=16  bin_pt=0  align_bp=on  overflow=[]  quantization=[]  XmcBlockStatus=1  maskContainerNames=tabcontainer1  block_type=logical  block_config=sysgen:Logical_config
  c_out : hdlBasic/Logical  logical_function=OR  inputs=3  en=off  latency=0  precision=Full  arith_type=Unsigned  n_bits=16  bin_pt=0  align_bp=on  overflow=[]  quantization=[]  XmcBlockStatus=1  maskContainerNames=tabcontainer1  block_type=logical  block_config=sysgen:Logical_config
  ALU_OUT (1 BIT) : Outport
  CARRY_OUT (1 BIT) : Outport  Port=2
  wires:
  Logical2/1 -> c_out/3
  A_INVERT (1 BIT)/1 -> Mux1/1
  c_out/1 -> CARRY_OUT (1 BIT)/1
  Sum/1 -> Mux/4
  CARRY_IN (1 BIT)/1 -> Inverter1/1, Logical5/1, Logical4/1, Logical1/1, Logical/1
  Mux2/1 -> Logical5/3, Logical6/3, Logical1/2, Logical2/2, Inverter9/1, Logical8/2, Logical3/2, Logical7/2
  B_INPUT (1 BIT)/1 -> Inverter3/1, Mux2/2
  Mux/1 -> ALU_OUT (1 BIT)/1
  Logical/1 -> c_out/1
  B_INVERT (1 BIT)/1 -> Mux2/1
  Logical6/1 -> Sum/3
  Mux1/1 -> Logical8/1, Logical7/1, Logical3/1, Inverter8/1, Logical5/2, Logical/2, Logical2/1, Logical9/2
  Logical5/1 -> Sum/4
  OP (2 BIT)/1 -> Mux/1
  Logical9/1 -> Sum/2
  Inverter1/1 -> Logical6/1, Logical9/1
  Inverter3/1 -> Mux2/3
  Inverter9/1 -> Logical9/3, Logical4/3
  A_INPUT (1 BIT)/1 -> Mux1/2, Inverter2/1
  Inverter2/1 -> Mux1/3
  Logical4/1 -> Sum/1
  Inverter8/1 -> Logical6/2, Logical4/2
  Logical3/1 -> Mux/2
  Logical7/1 -> Mux/3
  Logical1/1 -> c_out/2
  Logical8/1 -> Mux/5

== system ALU_04_SS/ALU_64_BITS/ALU_18 ==
  CARRY_IN (1 BIT) : Inport
  OP (2 BIT) : Inport  Port=2
  A_INVERT (1 BIT) : Inport  Port=3
  A_INPUT (1 BIT) : Inport  Port=4
  B_INVERT (1 BIT) : Inport  Port=5
  B_INPUT (1 BIT) : Inport  Port=6
  Inverter{1..3,8..9} (5 alike) : hdlBasic/Inverter  en=off  latency=0  XmcBlockStatus=1  maskContainerNames=group2  block_type=inv  block_config=sysgen:Inverter_config
  Logical{,1..3} (4 alike) : hdlBasic/Logical  logical_function=AND  inputs=2  en=off  latency=0  precision=Full  arith_type=Unsigned  n_bits=16  bin_pt=0  align_bp=on  overflow=[]  quantization=[]  XmcBlockStatus=1  maskContainerNames=tabcontainer1  block_type=logical  block_config=sysgen:Logical_config
  Logical{4..6,9} (4 alike) : hdlBasic/Logical  logical_function=AND  inputs=3  en=off  latency=0  precision=Full  arith_type=Unsigned  n_bits=16  bin_pt=0  align_bp=on  overflow=[]  quantization=[]  XmcBlockStatus=1  maskContainerNames=tabcontainer1  block_type=logical  block_config=sysgen:Logical_config
  Logical7 : hdlBasic/Logical  logical_function=OR  inputs=2  en=off  latency=0  precision=Full  arith_type=Unsigned  n_bits=16  bin_pt=0  align_bp=on  overflow=[]  quantization=[]  XmcBlockStatus=1  maskContainerNames=tabcontainer1  block_type=logical  block_config=sysgen:Logical_config
  Logical8 : hdlBasic/Logical  logical_function=XOR  inputs=2  en=off  latency=0  precision=Full  arith_type=Unsigned  n_bits=16  bin_pt=0  align_bp=on  overflow=[]  quantization=[]  XmcBlockStatus=1  maskContainerNames=tabcontainer1  block_type=logical  block_config=sysgen:Logical_config
  Mux : hdlBasic/Mux  inputs=4  en=off  latency=0  precision=Full  arith_type=Unsigned  n_bits=16  bin_pt=14  quantization=Truncate  overflow=Wrap  XmcBlockStatus=1  maskContainerNames=tabcontainer1  block_type=mux  block_config=sysgen:Mux_config
  Mux1 : hdlBasic/Mux  inputs=2  en=off  latency=0  precision=Full  arith_type=Unsigned  n_bits=16  bin_pt=14  quantization=Truncate  overflow=Wrap  XmcBlockStatus=1  maskContainerNames=tabcontainer1  block_type=mux  block_config=sysgen:Mux_config
  Mux2 : hdlBasic/Mux  inputs=2  en=off  latency=0  precision=Full  arith_type=Unsigned  n_bits=16  bin_pt=14  quantization=Truncate  overflow=Wrap  XmcBlockStatus=1  maskContainerNames=tabcontainer1  block_type=mux  block_config=sysgen:Mux_config
  Sum : hdlBasic/Logical  logical_function=OR  inputs=4  en=off  latency=0  precision=Full  arith_type=Unsigned  n_bits=16  bin_pt=0  align_bp=on  overflow=[]  quantization=[]  XmcBlockStatus=1  maskContainerNames=tabcontainer1  block_type=logical  block_config=sysgen:Logical_config
  c_out : hdlBasic/Logical  logical_function=OR  inputs=3  en=off  latency=0  precision=Full  arith_type=Unsigned  n_bits=16  bin_pt=0  align_bp=on  overflow=[]  quantization=[]  XmcBlockStatus=1  maskContainerNames=tabcontainer1  block_type=logical  block_config=sysgen:Logical_config
  ALU_OUT (1 BIT) : Outport
  CARRY_OUT (1 BIT) : Outport  Port=2
  wires:
  Logical2/1 -> c_out/3
  A_INVERT (1 BIT)/1 -> Mux1/1
  c_out/1 -> CARRY_OUT (1 BIT)/1
  Sum/1 -> Mux/4
  CARRY_IN (1 BIT)/1 -> Inverter1/1, Logical5/1, Logical4/1, Logical1/1, Logical/1
  Mux2/1 -> Logical5/3, Logical6/3, Logical1/2, Logical2/2, Inverter9/1, Logical8/2, Logical3/2, Logical7/2
  B_INPUT (1 BIT)/1 -> Inverter3/1, Mux2/2
  Mux/1 -> ALU_OUT (1 BIT)/1
  Logical/1 -> c_out/1
  B_INVERT (1 BIT)/1 -> Mux2/1
  Logical6/1 -> Sum/3
  Mux1/1 -> Logical8/1, Logical7/1, Logical3/1, Inverter8/1, Logical5/2, Logical/2, Logical2/1, Logical9/2
  Logical5/1 -> Sum/4
  OP (2 BIT)/1 -> Mux/1
  Logical9/1 -> Sum/2
  Inverter1/1 -> Logical6/1, Logical9/1
  Inverter3/1 -> Mux2/3
  Inverter9/1 -> Logical9/3, Logical4/3
  A_INPUT (1 BIT)/1 -> Mux1/2, Inverter2/1
  Inverter2/1 -> Mux1/3
  Logical4/1 -> Sum/1
  Inverter8/1 -> Logical6/2, Logical4/2
  Logical3/1 -> Mux/2
  Logical7/1 -> Mux/3
  Logical1/1 -> c_out/2
  Logical8/1 -> Mux/5

== system ALU_04_SS/ALU_64_BITS/ALU_19 ==
  CARRY_IN (1 BIT) : Inport
  OP (2 BIT) : Inport  Port=2
  A_INVERT (1 BIT) : Inport  Port=3
  A_INPUT (1 BIT) : Inport  Port=4
  B_INVERT (1 BIT) : Inport  Port=5
  B_INPUT (1 BIT) : Inport  Port=6
  Inverter{1..3,8..9} (5 alike) : hdlBasic/Inverter  en=off  latency=0  XmcBlockStatus=1  maskContainerNames=group2  block_type=inv  block_config=sysgen:Inverter_config
  Logical{,1..3} (4 alike) : hdlBasic/Logical  logical_function=AND  inputs=2  en=off  latency=0  precision=Full  arith_type=Unsigned  n_bits=16  bin_pt=0  align_bp=on  overflow=[]  quantization=[]  XmcBlockStatus=1  maskContainerNames=tabcontainer1  block_type=logical  block_config=sysgen:Logical_config
  Logical{4..6,9} (4 alike) : hdlBasic/Logical  logical_function=AND  inputs=3  en=off  latency=0  precision=Full  arith_type=Unsigned  n_bits=16  bin_pt=0  align_bp=on  overflow=[]  quantization=[]  XmcBlockStatus=1  maskContainerNames=tabcontainer1  block_type=logical  block_config=sysgen:Logical_config
  Logical7 : hdlBasic/Logical  logical_function=OR  inputs=2  en=off  latency=0  precision=Full  arith_type=Unsigned  n_bits=16  bin_pt=0  align_bp=on  overflow=[]  quantization=[]  XmcBlockStatus=1  maskContainerNames=tabcontainer1  block_type=logical  block_config=sysgen:Logical_config
  Logical8 : hdlBasic/Logical  logical_function=XOR  inputs=2  en=off  latency=0  precision=Full  arith_type=Unsigned  n_bits=16  bin_pt=0  align_bp=on  overflow=[]  quantization=[]  XmcBlockStatus=1  maskContainerNames=tabcontainer1  block_type=logical  block_config=sysgen:Logical_config
  Mux : hdlBasic/Mux  inputs=4  en=off  latency=0  precision=Full  arith_type=Unsigned  n_bits=16  bin_pt=14  quantization=Truncate  overflow=Wrap  XmcBlockStatus=1  maskContainerNames=tabcontainer1  block_type=mux  block_config=sysgen:Mux_config
  Mux1 : hdlBasic/Mux  inputs=2  en=off  latency=0  precision=Full  arith_type=Unsigned  n_bits=16  bin_pt=14  quantization=Truncate  overflow=Wrap  XmcBlockStatus=1  maskContainerNames=tabcontainer1  block_type=mux  block_config=sysgen:Mux_config
  Mux2 : hdlBasic/Mux  inputs=2  en=off  latency=0  precision=Full  arith_type=Unsigned  n_bits=16  bin_pt=14  quantization=Truncate  overflow=Wrap  XmcBlockStatus=1  maskContainerNames=tabcontainer1  block_type=mux  block_config=sysgen:Mux_config
  Sum : hdlBasic/Logical  logical_function=OR  inputs=4  en=off  latency=0  precision=Full  arith_type=Unsigned  n_bits=16  bin_pt=0  align_bp=on  overflow=[]  quantization=[]  XmcBlockStatus=1  maskContainerNames=tabcontainer1  block_type=logical  block_config=sysgen:Logical_config
  c_out : hdlBasic/Logical  logical_function=OR  inputs=3  en=off  latency=0  precision=Full  arith_type=Unsigned  n_bits=16  bin_pt=0  align_bp=on  overflow=[]  quantization=[]  XmcBlockStatus=1  maskContainerNames=tabcontainer1  block_type=logical  block_config=sysgen:Logical_config
  ALU_OUT (1 BIT) : Outport
  CARRY_OUT (1 BIT) : Outport  Port=2
  wires:
  Logical2/1 -> c_out/3
  A_INVERT (1 BIT)/1 -> Mux1/1
  c_out/1 -> CARRY_OUT (1 BIT)/1
  Sum/1 -> Mux/4
  CARRY_IN (1 BIT)/1 -> Inverter1/1, Logical5/1, Logical4/1, Logical1/1, Logical/1
  Mux2/1 -> Logical5/3, Logical6/3, Logical1/2, Logical2/2, Inverter9/1, Logical8/2, Logical3/2, Logical7/2
  B_INPUT (1 BIT)/1 -> Inverter3/1, Mux2/2
  Mux/1 -> ALU_OUT (1 BIT)/1
  Logical/1 -> c_out/1
  B_INVERT (1 BIT)/1 -> Mux2/1
  Logical6/1 -> Sum/3
  Mux1/1 -> Logical8/1, Logical7/1, Logical3/1, Inverter8/1, Logical5/2, Logical/2, Logical2/1, Logical9/2
  Logical5/1 -> Sum/4
  OP (2 BIT)/1 -> Mux/1
  Logical9/1 -> Sum/2
  Inverter1/1 -> Logical6/1, Logical9/1
  Inverter3/1 -> Mux2/3
  Inverter9/1 -> Logical9/3, Logical4/3
  A_INPUT (1 BIT)/1 -> Mux1/2, Inverter2/1
  Inverter2/1 -> Mux1/3
  Logical4/1 -> Sum/1
  Inverter8/1 -> Logical6/2, Logical4/2
  Logical3/1 -> Mux/2
  Logical7/1 -> Mux/3
  Logical1/1 -> c_out/2
  Logical8/1 -> Mux/5
